simulink model "HW2_PR1_integrated_PD"  (R2019a)
settings: Solver=VariableStepAuto  StartTime=0.0  StopTime=50  RelTol=1e-3
values from neighbouring files (symbols this model uses):
  A = [0 1 0 0;-(k_1+k_2)/m_1 -b/m_1 k_2/m_1 b/m_1;0 0 0 1;k_2/m_2 b/m_2 -k_2/m_2 -b/m_2]    [HW2_P2_a.m]    (also in HW2_P3_ab.m = [0 1; (-(k*L1*L1)/(m*L3*L3)) (-(c*L2*L2)/(m*L3*L3)) ]; HW2_Q1_parameters.m = 0.1)
  B = [0 0;k_1/m_1 -1/m_1;0 0;0 1/m_2]    [HW2_P2_a.m]    (also in HW2_P3_ab.m = [0;((k*L1)/(m*L3*L3))]; HW2_Q1_parameters.m = 0.1)
  b1 = 16    [HW2_Q1_parameters.m]
  c = 3    [HW2_P3_ab.m]    (also in HW2_Q1_parameters.m = 1; HW2_Q3_parameters.m)
  FL = 1    [HW2_Q1_parameters.m]
  h = 1    [HW2_Q1_parameters.m]
  k1 = 8    [HW2_Q1_parameters.m]
  ks = 10    [HW2_Q1_parameters.m]
  M = ks/wn^2    (= 0.0545218072481)    [HW2_Q1_parameters.m]
  m = 10    [HW2_P3_ab.m]    (also in HW2_Q1_parameters.m = 2; HW2_Q3_parameters.m)
  R = 10    [HW2_Q1_parameters.m]
  wd = ks/(zeta*2*sqrt(ks*M)- B- R*A*A)    [HW2_Q1_parameters.m]
settings Model: Creator=canba  LastModifiedBy=canba
settings SolverCC: AlgebraicLoopSolver=LineSearch

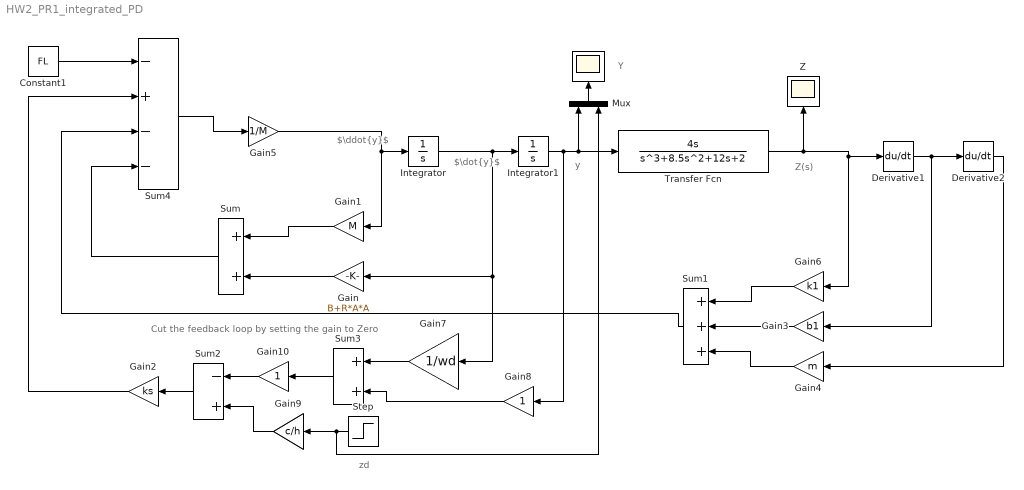
== system HW2_PR1_integrated_PD ==
  note: Y
  note: $\ddot{y}$
  note: Cut the feedback loop by setting the gain to Zero
  note: zd
  note: Z(s)
  note: y
  note: $\dot{y}$
  " " : Scope
  " Z" : Scope
  Constant1 : Constant  Value=FL
  Derivative1 : Derivative
  Derivative2 : Derivative
  Gain : Gain  Gain=B+R*A*A
  Gain1 : Gain  Gain=M
  Gain10 : Gain
  Gain2 : Gain  Gain=ks
  Gain3 : Gain  Gain=b1
  Gain4 : Gain  Gain=m
  Gain5 : Gain  Gain=1/M
  Gain6 : Gain  Gain=k1
  Gain7 : Gain  Gain=1/wd
  Gain8 : Gain
  Gain9 : Gain  Gain=c/h
  Integrator : Integrator
  Integrator1 : Integrator
  Mux : Mux  Inputs=2
  Step : Step  Time=10  SampleTime=0
  Sum : Sum
  Sum1 : Sum  Inputs=+++
  Sum2 : Sum  Inputs=-+
  Sum3 : Sum
  Sum4 : Sum  Inputs=-+--
  Transfer Fcn : TransferFcn  Numerator=[4 0]  Denominator=[1 8.5 12 2]
  wires:
  Integrator/1 -> Gain7/1, Gain/1, Integrator1/1
  Integrator1/1 -> Gain8/1, Mux/1, Transfer Fcn/1
  Transfer Fcn/1 -> " Z"/1, Derivative1/1, Gain6/1
  Gain/1 -> Sum/2
  Derivative1/1 -> Derivative2/1, Gain3/1
  Derivative2/1 -> Gain4/1
  Gain1/1 -> Sum/1
  Sum1/1 -> Sum4/3
  Gain7/1 -> Sum3/1
  Gain8/1 -> Sum3/2
  Sum3/1 -> Gain10/1
  Gain9/1 -> Sum2/2
  Sum2/1 -> Gain2/1
  Gain2/1 -> Sum4/2
  Constant1/1 -> Sum4/1
  Gain5/1 -> Gain1/1, Integrator/1
  Sum4/1 -> Gain5/1
  Sum/1 -> Sum4/4
  Gain3/1 -> Sum1/2
  Gain6/1 -> Sum1/1
  Gain4/1 -> Sum1/3
  Step/1 -> Mux/2, Gain9/1
  Gain10/1 -> Sum2/1
  Mux/1 -> " "/1
